simulink model "Model_G12_Numerical_Integration"  (Simulink 6.6)
settings: Solver=ode45  SolverMode=SingleTasking  StartTime=0.0  StopTime=T  RelTol=1e-3  AbsTol=1e-6
values from neighbouring files (symbols this model uses):
  damp = 2 * zeta * mass * w_nat    (= 1256.63706144)    [Pgm_G12_Num_Integration.m]
  dt = 0.01    [Pgm_G11_Superposition.m]    (also in Pgm_G12_Num_Integration.m; Pgm_G13_Frequency_Domain.m = 0.0625; Pgm_H2_Response_Gusts_Control.m = 0.001; Pgm_H3_Ase_Gusts_Pid.m = 0.001)
  mass = 1000    [Pgm_G11_Superposition.m]    (also in Pgm_G12_Num_Integration.m; Pgm_G13_Frequency_Domain.m)
  stiff = w_nat^2 * mass    (= 157913.670417)    [Pgm_G11_Superposition.m]    (also in Pgm_G12_Num_Integration.m; Pgm_G13_Frequency_Domain.m)
settings Model: Creator=Jan Wright  LastModifiedBy=Jan Wright
settings DataIOCC: LimitDataPoints=off
settings OptimizationCC: BlockReduction=off  BooleanDataType=off
settings DebuggingCC: SignalResolutionControl=TryResolveAllWithWarning  SolverPrmCheckMsg=none  MultiTaskDSMMsg=warning  MultiTaskCondExecSysMsg=none  StrictBusMsg=None
settings HardwareCC: TargetUnknown=on
settings RTWCC: IncludeERTFirstTime=on
settings GRTTargetCC: ModelReferenceCompliant=off  MatFileLogging=off

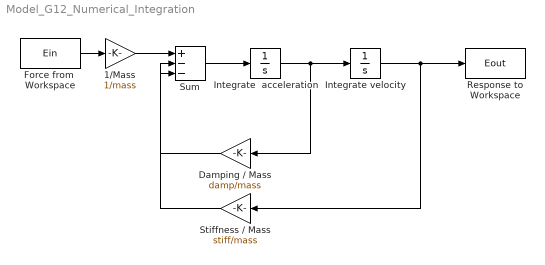
== system Model_G12_Numerical_Integration ==
  1/Mass : Gain  Gain=1/mass  SaturateOnIntegerOverflow=on
  Damping / Mass : Gain  Orientation=left  Gain=damp/mass  SaturateOnIntegerOverflow=on
  Force from  Workspace : FromWorkspace  VariableName=Ein  SampleTime=dt
  Integrate velocity : Integrator
  Integrate  acceleration : Integrator
  Response to Workspace : ToWorkspace  VariableName=Eout  SampleTime=dt  SaveFormat=Array
  Stiffness / Mass : Gain  Orientation=left  Gain=stiff/mass  SaturateOnIntegerOverflow=on
  Sum : Sum  Inputs=+--  SaturateOnIntegerOverflow=on  InputSameDT=on
  wires:
  Integrate  acceleration/1 -> Integrate velocity/1, Damping / Mass/1
  Integrate velocity/1 -> Stiffness / Mass/1, Response to Workspace/1
  Damping / Mass/1 -> Sum/3
  Stiffness / Mass/1 -> Sum/2
  1/Mass/1 -> Sum/1
  Sum/1 -> Integrate  acceleration/1
  Force from  Workspace/1 -> 1/Mass/1
